simulink model "BBBCSystem_NADR_F2PID"  (R2023b)
settings: Solver=ode3  StartTime=0.0  StopTime=25  FixedStep=0.01  RelTol=1e-3  EnableMultiTasking=on
values from neighbouring files (symbols this model uses):
  K0 = x(i,3)    [BCostPD.m]    (also in dataset.mat = 0.0001; initiateVars.m = 0.0001; system_workspace.mat = 0.0001; system_workspace_ayk.mat = 0.0001)
  K1 = x(i,4)    [BCostPD.m]    (also in dataset.mat = 0.1; initiateVars.m = 0.1; system_workspace.mat = 0.1; system_workspace_ayk.mat = 0.1)
  Kd = x(i,2)    [BCostPD.m]    (also in dataset.mat = 2; initiateVars.m = 2; system_workspace.mat = 2; system_workspace_ayk.mat = 2)
  Ke = x(i,1)    [BCostPD.m]    (also in dataset.mat = 1; initiateVars.m = 1; system_workspace.mat = 1; system_workspace_ayk.mat = 1)
undefined symbols (not defined in the file or in its folder): b0, beta_01, beta_02, beta_03, DiscIntNeverNeededParam, h, magnitude
libraries: simulink x4, fuzblock x2
settings Model: Creator=fd  LastModifiedBy=fethi
settings SolverCC: AlgebraicLoopSolver=TrustRegion  AutoInsertRateTranBlk=on
settings DataIOCC: LimitDataPoints=on  SaveFormat=Array  SignalLoggingSaveFormat=ModelDataLogs  ReturnWorkspaceOutputs=off
settings OptimizationCC: ExpressionDepthLimit=2147483647  LifeSpan=inf
settings DebuggingCC: UnderspecifiedInitializationDetection=Classic  MergeDetectMultiDrivingBlocksExec=none  SolverPrmCheckMsg=warning  MultiTaskDSMMsg=warning  MultiTaskCondExecSysMsg=none  FcnCallInpInsideContextMsg=warning  UnconnectedInputMsg=warning  UnconnectedOutputMsg=warning  UnconnectedLineMsg=warning  StateNameClashWarn=warning  SFUnexpectedBacktrackingDiag=warning  SFNoUnconditionalDefaultTransitionDiag=warning  SFExecutionAtInitializationDiag=none  ArithmeticOperatorsInVariantConditions=warning
settings HardwareCC: ProdBitPerPointer=32  ProdBitPerSizeT=32  ProdBitPerPtrDiffT=32  ProdLargestAtomicFloat=None  ProdIntDivRoundTo=Undefined  ProdEndianess=Unspecified  ProdWordSize=32  ProdHWDeviceType=32-bit Generic
settings ModelReferenceCC: PropagateSignalLabelsOutOfModel=off
settings SFSimCC: SimUseLocalCustomCode=off  CustomCodeUndefinedFunction=UseInterfaceOnly
settings RTWCC: RTWUseLocalCustomCode=off
settings CodeAppCC: StateflowObjectComments=on
settings GRTTargetCC: TargetLangStandard=C89/C90 (ANSI)  CombineOutputUpdateFcns=off  GRTInterface=on
settings ConfigComp: CovMetricSettings=dw  CovSaveCumulativeToWorkspaceVar=on  CovSaveSingleToWorkspaceVar=on  CovExternalEMLEnable=off

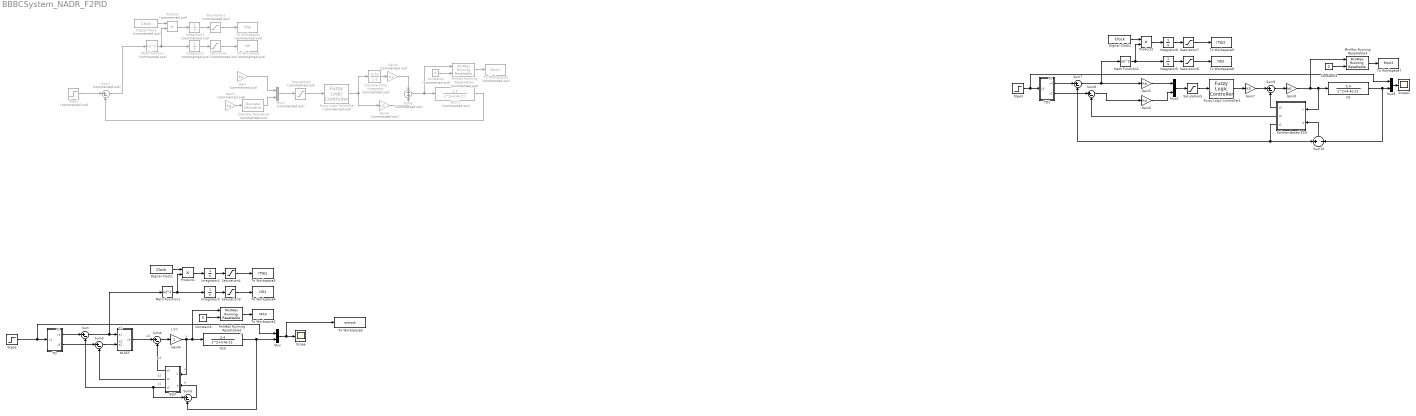
== system BBBCSystem_NADR_F2PID ==
  note: 1/b0
  note: v0
  note: u
  note: u
  note: y
  note: e1
  note: z1
  note: z3
  note: e2
  note: u0
  note: z2
  note: e
  note: v0
  Constant1 : Constant  Commented=on  Value=0
  Constant2 : Constant  Value=0
  Constant3 : Constant  Value=0
  Digital Clock : DigitalClock  Commented=on  SampleTime=0.01
  Digital Clock1 : DigitalClock  SampleTime=0.01
  Digital Clock2 : DigitalClock  SampleTime=0.01
  Discrete Derivative : simulink/Discrete/Discrete Derivative  Commented=on  gainval=1.0  ICPrevScaledInput=0.0  OutMin=[]  OutMax=[]  OutDataType=fixdt(1, 16)  OutScaling=2^-10  DoSatur=off
  Discrete-Time Integrator : DiscreteIntegrator  Commented=on  SampleTime=-1  ICPrevOutput=DiscIntNeverNeededParam  ICPrevScaledInput=DiscIntNeverNeededParam
  ESO : Subsystem  mask(ESO){h=0.01, beta_01=100, beta_02=300, beta_03=1000, b0=1}
      mask help: 这一部分（扩张状态观测器）的作用是得到系统状态变量的估计值及扩张状态的实时作用量。
      mask Display: disp('ESO');
  Fuzzy Logic Controller : fuzblock/Fuzzy Logic  Controller  Commented=on  FIS='fis2.fis'  OutputSampleNumber=101  DataType=double  FuzzifiedInputs=off  RuleFiringStrengths=off  RuleOutputs=off  AggregatedOutputs=off  SimulateUsing=Interpreted execution  OutOfRangeInputValueMessage=warning  NoRuleFiredMessage=warning  EmptyOutputFuzzySetMessage=warning
  Fuzzy Logic Controller1 : fuzblock/Fuzzy Logic  Controller  FIS='fis2.fis'  OutputSampleNumber=101  DataType=double  FuzzifiedInputs=off  RuleFiringStrengths=off  RuleOutputs=off  AggregatedOutputs=off  SimulateUsing=Interpreted execution  OutOfRangeInputValueMessage=warning  NoRuleFiredMessage=warning  EmptyOutputFuzzySetMessage=warning
  G1 : TransferFcn  Numerator=[2.4]  Denominator=[1 4.4 -11]
  G15 : TransferFcn  Numerator=[2.4]  Denominator=[1 4.4 -11]
  G15 1 : TransferFcn  Commented=on  Numerator=[2.4]  Denominator=[1 4.4 -11]
  Gain : Gain  Commented=on  Gain=Ke
  Gain1 : Gain  Commented=on  Gain=Kd
  Gain2 : Gain  Commented=on  Gain=K0
  Gain3 : Gain  Commented=on  Gain=K1
  Gain4 : Gain
  Gain5 : Gain  Gain=Ke
  Gain6 : Gain  Gain=Kd
  Gain7 : Gain  Gain=K0
  Gain9 : Gain  Gain=b0
  Integrator1 : Integrator  Commented=on
  Integrator2 : Integrator  Commented=on
  Integrator{3..6} (4 alike) : Integrator
  Kalman-Based ESO : Subsystem
  Math Function : Math  Commented=on  Operator=magnitude^2  SignedPower=on
  Math Function1 : Math  Operator=magnitude^2  SignedPower=on
  Math Function2 : Math  Operator=magnitude^2  SignedPower=on
  MinMax Running Resettable1 : simulink/Math Operations/MinMax Running Resettable  Commented=on  Function=max  vinit=0
  MinMax Running Resettable2 : simulink/Math Operations/MinMax Running Resettable  Function=max  vinit=0
  MinMax Running Resettable3 : simulink/Math Operations/MinMax Running Resettable  Function=max  vinit=0
  Mux : Mux  Inputs=2
  Mux1 : Mux  Commented=on  Inputs=2
  Mux2 : Mux  Inputs=2
  Mux3 : Mux  Inputs=2
  NLSEF : Subsystem  mask(NLSEF){c=0.3, r=5, h1=0.03}
      mask help: 非线性状态误差反馈律是把跟踪微分器产生的跟踪信号和微分信号与扩张状态观测器得到的系统的状态估计通过非线性函数进行适当组合，作为被控对象的控制量。
      mask Display: disp('NLSEF');
  Product : Product  Commented=on  RndMeth=Zero
  Product1 : Product  RndMeth=Zero
  Product2 : Product  RndMeth=Zero
  Saturation : Saturate  Commented=on  UpperLimit=800
  Saturation1 : Saturate  Commented=on  UpperLimit=800
  Saturation2 : Saturate  Commented=on  UpperLimit=1  LowerLimit=-1
  Saturation{3..4,6..7} (4 alike) : Saturate  UpperLimit=800
  Saturation5 : Saturate  UpperLimit=1  LowerLimit=-1
  Scope : Scope
  Scope1 : Scope
  Step1 : Step  Commented=on  Time=0  SampleTime=0.01
  Step2 : Step  Time=0  SampleTime=0.05
  Step3 : Step  Time=0  SampleTime=0.05
  Sum{,3..5,7..9} (7 alike) : Sum  Inputs=|+-
  Sum1 : Sum  Commented=on  Inputs=|+-
  Sum10 : Sum  Inputs=+||-
  Sum2 : Sum  Commented=on  Inputs=+|+
  TD : Subsystem  mask(TD){r0=2.0, h=0.01}
      mask help: 跟踪微分器为系统输入安排过渡过程，得到光滑的输入信号以及输入信号的微分信号。
      mask Display: disp('TD');
  TD1 : Subsystem  mask(TD){r0=2.0, h=0.01}
      mask help: 跟踪微分器为系统输入安排过渡过程，得到光滑的输入信号以及输入信号的微分信号。
      mask Display: disp('TD');
  To Workspace : ToWorkspace  Commented=on  VariableName=ISE  SampleTime=-1
  To Workspace1 : ToWorkspace  Commented=on  VariableName=ITSE  SampleTime=-1
  To Workspace2 : ToWorkspace  VariableName=MAX  SampleTime=-1
  To Workspace3 : ToWorkspace  Commented=on  VariableName=MAX1  SampleTime=-1
  To Workspace4 : ToWorkspace  VariableName=ISE1  SampleTime=-1
  To Workspace5 : ToWorkspace  VariableName=ITSE1  SampleTime=-1
  To Workspace6 : ToWorkspace  VariableName=simout  SaveFormat=Timeseries  SampleTime=-1
  To Workspace7 : ToWorkspace  VariableName=MAX2  SampleTime=-1
  To Workspace8 : ToWorkspace  VariableName=ISE2  SampleTime=-1
  To Workspace9 : ToWorkspace  VariableName=ITSE2  SampleTime=-1
  wires:
  Integrator1/1 -> Saturation/1
  Math Function/1 -> Product/2, Integrator1/1
  Saturation/1 -> To Workspace/1
  Digital Clock/1 -> Product/1
  Product/1 -> Integrator2/1
  Integrator2/1 -> Saturation1/1
  Saturation1/1 -> To Workspace1/1
  Discrete Derivative/1 -> Mux1/2
  Gain3/1 -> Sum2/1
  Gain2/1 -> Sum2/2
  Gain1/1 -> Discrete Derivative/1
  Fuzzy Logic Controller/1 -> Gain2/1, Discrete-Time Integrator/1
  Discrete-Time Integrator/1 -> Gain3/1
  Step1/1 -> Sum1/1
  Gain/1 -> Mux1/1
  G15 1/1 -> Sum1/2
  Constant1/1 -> MinMax Running Resettable1/2
  MinMax Running Resettable1/1 -> To Workspace3/1
  Sum2/1 -> MinMax Running Resettable1/1, G15 1/1
  Sum1/1 -> Math Function/1
  Mux1/1 -> Saturation2/1
  Saturation2/1 -> Fuzzy Logic Controller/1
  ESO/2(z2) -> Sum3/2
  ESO/3(z1) -> Sum5/1, Sum/2
  Sum5/1 -> ESO/2(e)
  ESO/1(z3) -> Sum4/2
  TD/2(v5) -> Sum3/1
  Sum4/1 -> Gain4/1
  NLSEF/1(u0) -> Sum4/1
  Sum3/1 -> NLSEF/2(e2)
  TD/1(v4) -> Sum/1
  Sum/1 -> Math Function1/1, NLSEF/1(e1)
  G15/1 -> Mux/2, Sum5/2
  Gain4/1 -> MinMax Running Resettable2/1, G15/1, ESO/1(u)
  MinMax Running Resettable2/1 -> To Workspace2/1
  Constant2/1 -> MinMax Running Resettable2/2
  Step2/1 -> Mux/1, TD/1(v3)
  Mux/1 -> To Workspace6/1, Scope/1
  Saturation4/1 -> To Workspace5/1
  Integrator4/1 -> Saturation4/1
  Product1/1 -> Integrator4/1
  Digital Clock1/1 -> Product1/1
  Saturation3/1 -> To Workspace4/1
  Math Function1/1 -> Integrator3/1, Product1/2
  Integrator3/1 -> Saturation3/1
  Saturation5/1 -> Fuzzy Logic Controller1/1
  Integrator6/1 -> Saturation7/1
  Digital Clock2/1 -> Product2/1
  Saturation6/1 -> To Workspace8/1
  Product2/1 -> Integrator6/1
  Saturation7/1 -> To Workspace9/1
  G1/1 -> Mux3/2, Sum10/2
  Gain9/1 -> Kalman-Based ESO/1(u), G1/1, MinMax Running Resettable3/1
  Step3/1 -> Mux3/1, TD1/1(v3)
  Math Function2/1 -> Integrator5/1, Product2/2
  Integrator5/1 -> Saturation6/1
  MinMax Running Resettable3/1 -> To Workspace7/1
  Kalman-Based ESO/3(z1) -> Sum7/2, Sum10/1
  Sum10/1 -> Kalman-Based ESO/2(e)
  Sum9/1 -> Gain9/1
  TD1/2(v5) -> Sum8/1
  Sum7/1 -> Gain5/1, Math Function2/1
  Kalman-Based ESO/1(z3) -> Sum9/2
  Kalman-Based ESO/2(z2) -> Sum8/2
  Mux3/1 -> Scope1/1
  TD1/1(v4) -> Sum7/1
  Constant3/1 -> MinMax Running Resettable3/2
  Mux2/1 -> Saturation5/1
  Gain5/1 -> Mux2/1
  Sum8/1 -> Gain6/1
  Gain6/1 -> Mux2/2
  Gain7/1 -> Sum9/1
  Fuzzy Logic Controller1/1 -> Gain7/1

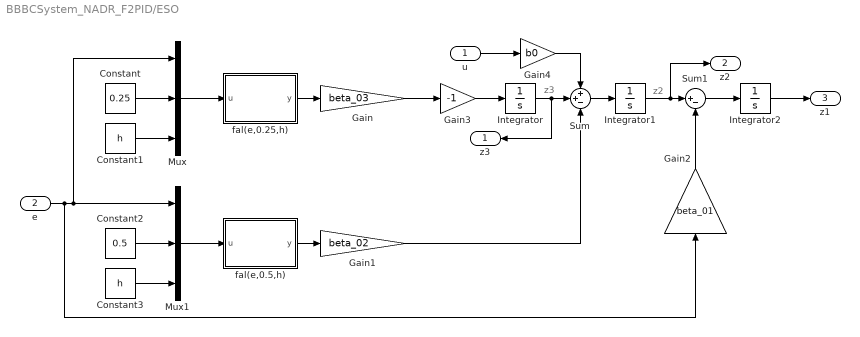
== system BBBCSystem_NADR_F2PID/ESO ==
  note: z2
  note: z3
  u : Inport
  e : Inport  Port=2
  Constant : Constant  Value=0.25
  Constant1 : Constant  Value=h
  Constant2 : Constant  Value=0.5
  Constant3 : Constant  Value=h
  Gain : Gain  Gain=beta_03
  Gain1 : Gain  Gain=beta_02
  Gain2 : Gain  Gain=beta_01
  Gain3 : Gain  Gain=-1
  Gain4 : Gain  Gain=b0
  Integrator : Integrator
  Integrator1 : Integrator
  Integrator2 : Integrator
  Mux : Mux  Inputs=[1 1 1]
  Mux1 : Mux  Inputs=[1 1 1]
  Sum : Sum  Inputs=++-
  Sum1 : Sum  Inputs=|+-
  fal(e,0.25,h) : MATLAB Function  TreatAsAtomicUnit=on
  fal(e,0.5,h) : MATLAB Function  TreatAsAtomicUnit=on
  z3 : Outport
  z2 : Outport  Port=2
  z1 : Outport  Port=3
  wires:
  Mux1/1 -> fal(e,0.5,h)/1(u)
  Mux/1 -> fal(e,0.25,h)/1(u)
  e/1 -> Gain2/1, Mux/1, Mux1/1
  Constant1/1 -> Mux/3
  Sum/1 -> Integrator1/1
  Gain2/1 -> Sum1/2
  Constant2/1 -> Mux1/2
  Gain4/1 -> Sum/1
  Integrator/1 -> z3/1, Sum/2
  fal(e,0.25,h)/1(y) -> Gain/1
  u/1 -> Gain4/1
  Gain1/1 -> Sum/3
  Constant3/1 -> Mux1/3
  Constant/1 -> Mux/2
  Integrator1/1 -> z2/1, Sum1/1
  Gain/1 -> Gain3/1
  Gain3/1 -> Integrator/1
  Sum1/1 -> Integrator2/1
  fal(e,0.5,h)/1(y) -> Gain1/1
  Integrator2/1 -> z1/1

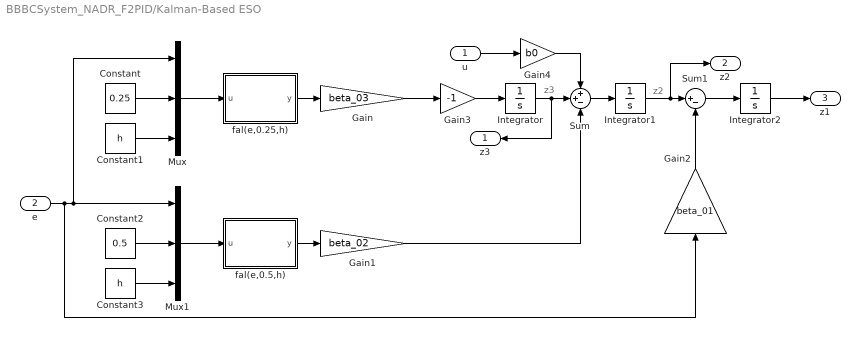
== system BBBCSystem_NADR_F2PID/Kalman-Based ESO ==
  note: z2
  note: z3
  u : Inport
  e : Inport  Port=2
  Constant : Constant  Value=0.25
  Constant1 : Constant  Value=h
  Constant2 : Constant  Value=0.5
  Constant3 : Constant  Value=h
  Gain : Gain  Gain=beta_03
  Gain1 : Gain  Gain=beta_02
  Gain2 : Gain  Gain=beta_01
  Gain3 : Gain  Gain=-1
  Gain4 : Gain  Gain=b0
  Integrator : Integrator
  Integrator1 : Integrator
  Integrator2 : Integrator
  Mux : Mux  Inputs=[1 1 1]
  Mux1 : Mux  Inputs=[1 1 1]
  Sum : Sum  Inputs=++-
  Sum1 : Sum  Inputs=|+-
  fal(e,0.25,h) : MATLAB Function  TreatAsAtomicUnit=on
  fal(e,0.5,h) : MATLAB Function  TreatAsAtomicUnit=on
  z3 : Outport
  z2 : Outport  Port=2
  z1 : Outport  Port=3
  wires:
  Constant/1 -> Mux/2
  fal(e,0.5,h)/1(y) -> Gain1/1
  Gain4/1 -> Sum/1
  Mux1/1 -> fal(e,0.5,h)/1(u)
  Integrator2/1 -> z1/1
  Gain1/1 -> Sum/3
  fal(e,0.25,h)/1(y) -> Gain/1
  e/1 -> Gain2/1, Mux/1, Mux1/1
  Integrator/1 -> z3/1, Sum/2
  u/1 -> Gain4/1
  Constant2/1 -> Mux1/2
  Gain3/1 -> Integrator/1
  Gain/1 -> Gain3/1
  Constant3/1 -> Mux1/3
  Integrator1/1 -> z2/1, Sum1/1
  Constant1/1 -> Mux/3
  Sum/1 -> Integrator1/1
  Mux/1 -> fal(e,0.25,h)/1(u)
  Gain2/1 -> Sum1/2
  Sum1/1 -> Integrator2/1

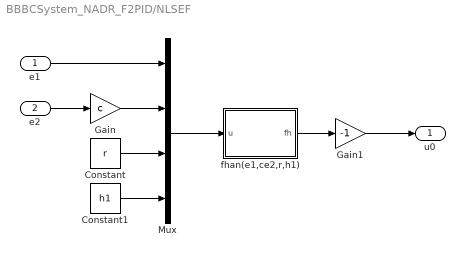
== system BBBCSystem_NADR_F2PID/NLSEF ==
  e1 : Inport
  e2 : Inport  Port=2
  Constant : Constant  Value=r
  Constant1 : Constant  Value=h1
  Gain : Gain  Gain=c
  Gain1 : Gain  Gain=-1
  Mux : Mux  Inputs=[1 1 1 1]
  fhan(e1,ce2,r,h1) : MATLAB Function  TreatAsAtomicUnit=on
  u0 : Outport
  wires:
  Mux/1 -> fhan(e1,ce2,r,h1)/1(u)
  Constant/1 -> Mux/3
  e2/1 -> Gain/1
  e1/1 -> Mux/1
  Constant1/1 -> Mux/4
  fhan(e1,ce2,r,h1)/1(fh) -> Gain1/1
  Gain1/1 -> u0/1
  Gain/1 -> Mux/2

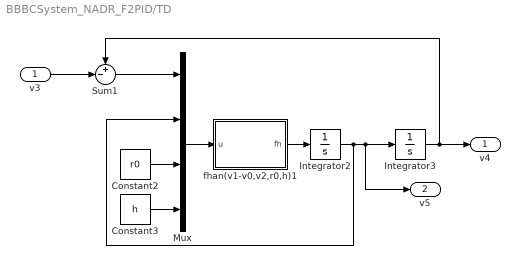
== system BBBCSystem_NADR_F2PID/TD ==
  v3 : Inport
  Constant2 : Constant  Value=r0
  Constant3 : Constant  Value=h
  Integrator2 : Integrator
  Integrator3 : Integrator
  Mux : Mux  Inputs=[1 1 1 1]
  Sum1 : Sum  Inputs=+-|
  fhan(v1-v0,v2,r0,h)1 : MATLAB Function  TreatAsAtomicUnit=on
  v4 : Outport
  v5 : Outport  Port=2
  wires:
  Constant2/1 -> Mux/3
  Mux/1 -> fhan(v1-v0,v2,r0,h)1/1(u)
  v3/1 -> Sum1/2
  fhan(v1-v0,v2,r0,h)1/1(fh) -> Integrator2/1
  Integrator2/1 -> v5/1, Integrator3/1, Mux/2
  Sum1/1 -> Mux/1
  Constant3/1 -> Mux/4
  Integrator3/1 -> v4/1, Sum1/1

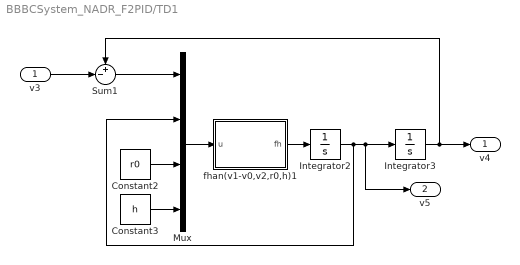
== system BBBCSystem_NADR_F2PID/TD1 ==
  v3 : Inport
  Constant2 : Constant  Value=r0
  Constant3 : Constant  Value=h
  Integrator2 : Integrator
  Integrator3 : Integrator
  Mux : Mux  Inputs=[1 1 1 1]
  Sum1 : Sum  Inputs=+-|
  fhan(v1-v0,v2,r0,h)1 : MATLAB Function  TreatAsAtomicUnit=on
  v4 : Outport
  v5 : Outport  Port=2
  wires:
  Constant2/1 -> Mux/3
  Mux/1 -> fhan(v1-v0,v2,r0,h)1/1(u)
  v3/1 -> Sum1/2
  fhan(v1-v0,v2,r0,h)1/1(fh) -> Integrator2/1
  Integrator2/1 -> v5/1, Integrator3/1, Mux/2
  Sum1/1 -> Mux/1
  Constant3/1 -> Mux/4
  Integrator3/1 -> v4/1, Sum1/1

== matlab function BBBCSystem_NADR_F2PID/ESO/fal(e,0.25,h) ==
  data: u input; y output
function y = fcn(u)

x = u(1);
alpha = u(2);
d = u(3);

if abs(x) <= d
    y = x / (d ^ (1 - alpha));
else 
    y = abs(x) ^ alpha * sign(x);
end

== matlab function BBBCSystem_NADR_F2PID/ESO/fal(e,0.5,h) ==
  data: u input; y output
function y = fcn(u)

x = u(1);
alpha = u(2);
d = u(3);

if abs(x) <= d
    y = x / (d ^ (1 - alpha));
else 
    y = abs(x) ^ alpha * sign(x);
end

== matlab function BBBCSystem_NADR_F2PID/TD/fhan(v1-v0,v2,r0,h)1 ==
  data: u input; fh output
function fh = fcn(u)

x1 = u(1);
x2 = u(2);
r = u(3);
h = u(4);

d = r * h * h;
a0 = h * x2;
y = x1 + a0;
a1 = sqrt(d * (d + 8 * abs(y)));
a2 = a0 + sign(y) * (a1 - d) / 2;
sy = (sign(y + d) - sign(y - d)) / 2;
a = (a0 + y - a2) * sy + a2;
sa = (sign(a + d) - sign(a - d)) / 2;

fh = -r * (a / d - sign(a)) * sa - r * sign(a);

== matlab function BBBCSystem_NADR_F2PID/Kalman-Based ESO/fal(e,0.25,h) ==
  data: u input; y output
function y = fcn(u)

x = u(1);
alpha = u(2);
d = u(3);

if abs(x) <= d
    y = x / (d ^ (1 - alpha));
else 
    y = abs(x) ^ alpha * sign(x);
end

== matlab function BBBCSystem_NADR_F2PID/TD1/fhan(v1-v0,v2,r0,h)1 ==
  data: u input; fh output
function fh = fcn(u)

x1 = u(1);
x2 = u(2);
r = u(3);
h = u(4);

d = r * h * h;
a0 = h * x2;
y = x1 + a0;
a1 = sqrt(d * (d + 8 * abs(y)));
a2 = a0 + sign(y) * (a1 - d) / 2;
sy = (sign(y + d) - sign(y - d)) / 2;
a = (a0 + y - a2) * sy + a2;
sa = (sign(a + d) - sign(a - d)) / 2;

fh = -r * (a / d - sign(a)) * sa - r * sign(a);

== matlab function BBBCSystem_NADR_F2PID/Kalman-Based ESO/fal(e,0.5,h) ==
  data: u input; y output
function y = fcn(u)

x = u(1);
alpha = u(2);
d = u(3);

if abs(x) <= d
    y = x / (d ^ (1 - alpha));
else 
    y = abs(x) ^ alpha * sign(x);
end

== matlab function BBBCSystem_NADR_F2PID/NLSEF/fhan(e1,ce2,r,h1) ==
  data: u input; fh output
function fh = fcn(u)

x1 = u(1);
x2 = u(2);
r = u(3);
h = u(4);

d = r * h * h;
a0 = h * x2;
y = x1 + a0;
a1 = sqrt(d * (d + 8 * abs(y)));
a2 = a0 + sign(y) * (a1 - d) / 2;
sy = (sign(y + d) - sign(y - d)) / 2;
a = (a0 + y - a2) * sy + a2;
sa = (sign(a + d) - sign(a - d)) / 2;

fh = -r * (a / d - sign(a)) * sa - r * sign(a);
